simulink model "canrx_0x6A2"  (R2022b)
settings: configuration reference "SLDD_CFG" (kept outside this file)
values from neighbouring files (symbols this model uses):
  K_CAN_GMLAN_RX_DEFAULT_ANMSIG_VCM_CAN02 = 0.0    [canrx_0x6A2.sldd]
  K_CAN_GMLAN_RX_INVALID_SELECT = 0.0    [canrx_0x6A2.sldd]
  K_CAN_RQST_SEL_2 = 0.0    [canrx_0x6A2.sldd]
  K_RQST_DRCT_2 = 0.0    [canrx_0x6A2.sldd]
libraries: user_lib x1, simulink x1
settings Model: DataDictionary=canrx_0x6A2.sldd  Creator=Castiel  LastModifiedBy=Castiel
settings ConfigSetRef: SourceName=SLDD_CFG

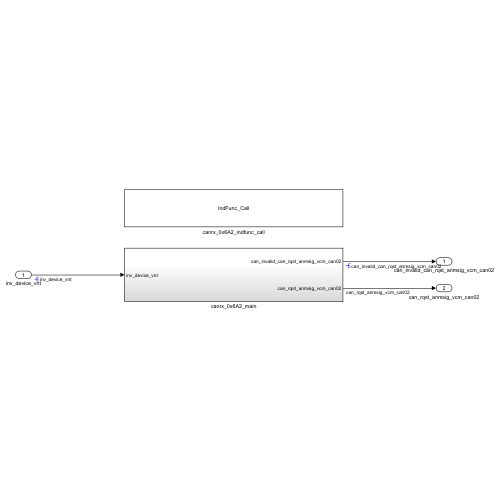
[thumbnail: Simulink's stored preview of the top-level diagram]
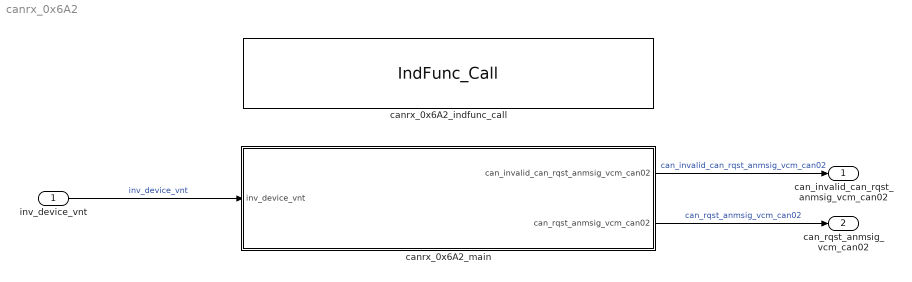
== system canrx_0x6A2 ==
  inv_device_vnt : Inport
  canrx_0x6A2_indfunc_call : user_lib/IndFunc_Call  siggroupIndex=Test  canid=6A2  signalTable={'UW','IFLayer_rx_anmsig_vcm_can02','SYCANC_COM2AP_6A2_rx_anmsig_vcm_can02'}  timeoutflag=off  extendid=off
      settings: SourceProductName=User Defined for IFLayer
  canrx_0x6A2_main : Subsystem
  can_invalid_can_rqst_anmsig_vcm_can02 : Outport
  can_rqst_anmsig_vcm_can02 : Outport  Port=2
  wires:
  inv_device_vnt/1 -> canrx_0x6A2_main/1(inv_device_vnt)  "inv_device_vnt"
  canrx_0x6A2_main/1(can_invalid_can_rqst_anmsig_vcm_can02) -> can_invalid_can_rqst_anmsig_vcm_can02/1  "can_invalid_can_rqst_anmsig_vcm_can02"
  canrx_0x6A2_main/2(can_rqst_anmsig_vcm_can02) -> can_rqst_anmsig_vcm_can02/1  "can_rqst_anmsig_vcm_can02"

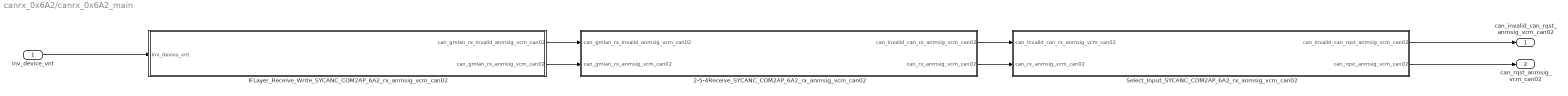
== system canrx_0x6A2/canrx_0x6A2_main ==
  inv_device_vnt : Inport
  2-5-4Receive_SYCANC_COM2AP_6A2_rx_anmsig_vcm_can02 : Subsystem  TreatAsAtomicUnit=on
      settings: RTWSystemCode=Nonreusable function
  IFLayer_Receive_Write_SYCANC_COM2AP_6A2_rx_anmsig_vcm_can02 : Subsystem  TreatAsAtomicUnit=on
      settings: RTWSystemCode=Nonreusable function
  Select_Input_SYCANC_COM2AP_6A2_rx_anmsig_vcm_can02 : Subsystem  TreatAsAtomicUnit=on
      settings: RTWSystemCode=Nonreusable function
  can_invalid_can_rqst_anmsig_vcm_can02 : Outport
  can_rqst_anmsig_vcm_can02 : Outport  Port=2
  wires:
  IFLayer_Receive_Write_SYCANC_COM2AP_6A2_rx_anmsig_vcm_can02/2(can_gmlan_rx_anmsig_vcm_can02) -> 2-5-4Receive_SYCANC_COM2AP_6A2_rx_anmsig_vcm_can02/2(can_gmlan_rx_anmsig_vcm_can02)
  IFLayer_Receive_Write_SYCANC_COM2AP_6A2_rx_anmsig_vcm_can02/1(can_gmlan_rx_invalid_anmsig_vcm_can02) -> 2-5-4Receive_SYCANC_COM2AP_6A2_rx_anmsig_vcm_can02/1(can_gmlan_rx_invalid_anmsig_vcm_can02)
  2-5-4Receive_SYCANC_COM2AP_6A2_rx_anmsig_vcm_can02/1(can_invalid_can_rx_anmsig_vcm_can02) -> Select_Input_SYCANC_COM2AP_6A2_rx_anmsig_vcm_can02/1(can_invalid_can_rx_anmsig_vcm_can02)
  2-5-4Receive_SYCANC_COM2AP_6A2_rx_anmsig_vcm_can02/2(can_rx_anmsig_vcm_can02) -> Select_Input_SYCANC_COM2AP_6A2_rx_anmsig_vcm_can02/2(can_rx_anmsig_vcm_can02)
  inv_device_vnt/1 -> IFLayer_Receive_Write_SYCANC_COM2AP_6A2_rx_anmsig_vcm_can02/1(inv_device_vnt)
  Select_Input_SYCANC_COM2AP_6A2_rx_anmsig_vcm_can02/1(can_invalid_can_rqst_anmsig_vcm_can02) -> can_invalid_can_rqst_anmsig_vcm_can02/1
  Select_Input_SYCANC_COM2AP_6A2_rx_anmsig_vcm_can02/2(can_rqst_anmsig_vcm_can02) -> can_rqst_anmsig_vcm_can02/1

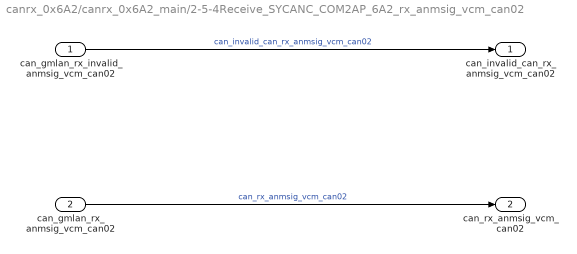
== system canrx_0x6A2/canrx_0x6A2_main/2-5-4Receive_SYCANC_COM2AP_6A2_rx_anmsig_vcm_can02 ==
  can_gmlan_rx_invalid_anmsig_vcm_can02 : Inport
  can_gmlan_rx_anmsig_vcm_can02 : Inport  Port=2
  can_invalid_can_rx_anmsig_vcm_can02 : Outport
  can_rx_anmsig_vcm_can02 : Outport  Port=2
  wires:
  can_gmlan_rx_anmsig_vcm_can02/1 -> can_rx_anmsig_vcm_can02/1  "can_rx_anmsig_vcm_can02"
  can_gmlan_rx_invalid_anmsig_vcm_can02/1 -> can_invalid_can_rx_anmsig_vcm_can02/1  "can_invalid_can_rx_anmsig_vcm_can02"

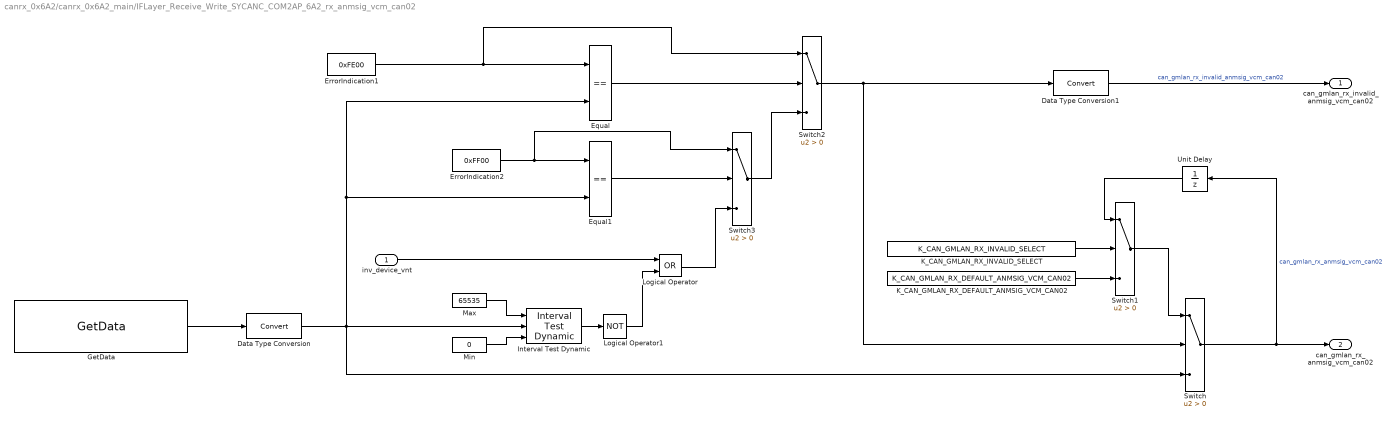
== system canrx_0x6A2/canrx_0x6A2_main/IFLayer_Receive_Write_SYCANC_COM2AP_6A2_rx_anmsig_vcm_can02 ==
  inv_device_vnt : Inport
  Data Type Conversion : DataTypeConversion  ConvertRealWorld=Stored Integer (SI)  SaturateOnIntegerOverflow=off  RndMeth=Floor
  Data Type Conversion1 : DataTypeConversion  ConvertRealWorld=Stored Integer (SI)  SaturateOnIntegerOverflow=off  RndMeth=Floor
  Equal : RelationalOperator  Operator===  OutDataTypeStr=boolean  RndMeth=Simplest  InputSameDT=off
  Equal1 : RelationalOperator  Operator===  OutDataTypeStr=boolean  RndMeth=Simplest  InputSameDT=off
  ErrorIndication1 : Constant  Value=0xFE00  OutDataTypeStr=Inherit: Inherit via back propagation
  ErrorIndication2 : Constant  Value=0xFF00  OutDataTypeStr=Inherit: Inherit via back propagation
  GetData : S-Function  FunctionName=GetData  Parameters=interface,signalType  SFunctionDeploymentMode=off  EnableBusSupport=off  mask{interface=SYCANC_COM2AP_6A2_rx_anmsig_vcm_can02, signalType=UW}
      mask prompts: signalType "Signal Type"
      mask TypeOptions signalType: UB | SB | UW | SW | UD | SD
      mask DialogControl Container4 Prompt: Singal Parameter
      mask Display:
      | interfaceName = get_param(gcbh, "interface");
      | s = strcat(interfaceName);
      | disp(s);
  Interval Test Dynamic : simulink/Logic and Bit Operations/Interval Test Dynamic  IntervalClosedRight=on  IntervalClosedLeft=on  OutDataTypeStr=boolean
  K_CAN_GMLAN_RX_DEFAULT_ANMSIG_VCM_CAN02 : Constant  Value=K_CAN_GMLAN_RX_DEFAULT_ANMSIG_VCM_CAN02  OutDataTypeStr=Inherit: Inherit via back propagation
  K_CAN_GMLAN_RX_INVALID_SELECT : Constant  Value=K_CAN_GMLAN_RX_INVALID_SELECT  OutDataTypeStr=Inherit: Inherit via back propagation
  Logical Operator : Logic  Operator=OR  AllPortsSameDT=off  OutDataTypeStr=boolean
  Logical Operator1 : Logic  Operator=NOT  AllPortsSameDT=off  OutDataTypeStr=boolean
  Max : Constant  Value=65535  OutDataTypeStr=Inherit: Inherit via back propagation
  Min : Constant  Value=0  OutDataTypeStr=Inherit: Inherit via back propagation
  Switch{,1..3} (4 alike) : Switch  Criteria=u2 > Threshold  SaturateOnIntegerOverflow=off  InputSameDT=off
  Unit Delay : UnitDelay  SampleTime=-1  HasFrameUpgradeWarning=on
  can_gmlan_rx_invalid_anmsig_vcm_can02 : Outport
  can_gmlan_rx_anmsig_vcm_can02 : Outport  Port=2
  wires:
  Switch1/1 -> Switch/1
  Unit Delay/1 -> Switch1/1
  inv_device_vnt/1 -> Logical Operator/1
  K_CAN_GMLAN_RX_DEFAULT_ANMSIG_VCM_CAN02/1 -> Switch1/3
  Max/1 -> Interval Test Dynamic/1
  Min/1 -> Interval Test Dynamic/3
  Switch/1 -> Unit Delay/1, can_gmlan_rx_anmsig_vcm_can02/1  "can_gmlan_rx_anmsig_vcm_can02"
  K_CAN_GMLAN_RX_INVALID_SELECT/1 -> Switch1/2
  Data Type Conversion1/1 -> can_gmlan_rx_invalid_anmsig_vcm_can02/1  "can_gmlan_rx_invalid_anmsig_vcm_can02"
  Logical Operator1/1 -> Logical Operator/2
  Interval Test Dynamic/1 -> Logical Operator1/1
  Equal/1 -> Switch2/2
  Switch2/1 -> Data Type Conversion1/1, Switch/2
  GetData/1 -> Data Type Conversion/1
  Equal1/1 -> Switch3/2
  Logical Operator/1 -> Switch3/3
  Switch3/1 -> Switch2/3
  Data Type Conversion/1 -> Equal1/2, Equal/2, Interval Test Dynamic/2, Switch/3
  ErrorIndication1/1 -> Switch2/1, Equal/1
  ErrorIndication2/1 -> Switch3/1, Equal1/1

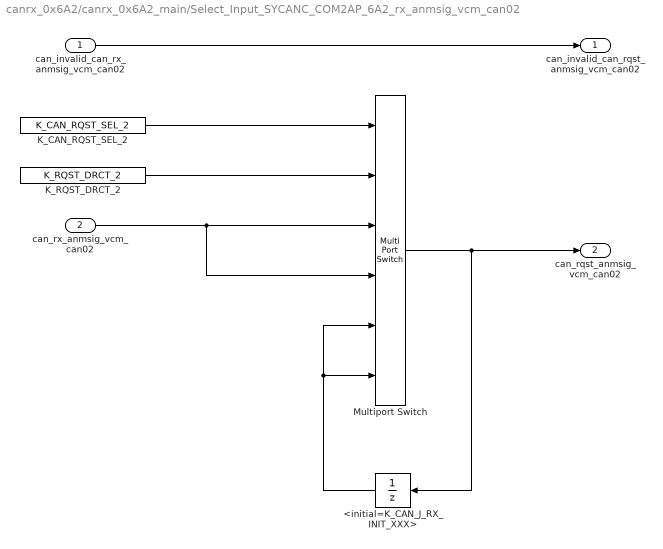
== system canrx_0x6A2/canrx_0x6A2_main/Select_Input_SYCANC_COM2AP_6A2_rx_anmsig_vcm_can02 ==
  can_invalid_can_rx_anmsig_vcm_can02 : Inport
  can_rx_anmsig_vcm_can02 : Inport  Port=2
  <initial=K_CAN_J_RX_INIT_XXX> : UnitDelay  SampleTime=-1  HasFrameUpgradeWarning=on
  K_CAN_RQST_SEL_2 : Constant  Value=K_CAN_RQST_SEL_2
  K_RQST_DRCT_2 : Constant  Value=K_RQST_DRCT_2
  Multiport Switch : MultiPortSwitch  DataPortOrder=Zero-based contiguous  Inputs=5  zeroidx=on  SaturateOnIntegerOverflow=off  InputSameDT=off
  can_invalid_can_rqst_anmsig_vcm_can02 : Outport
  can_rqst_anmsig_vcm_can02 : Outport  Port=2
  wires:
  K_CAN_RQST_SEL_2/1 -> Multiport Switch/1
  <initial=K_CAN_J_RX_INIT_XXX>/1 -> Multiport Switch/6, Multiport Switch/5
  Multiport Switch/1 -> can_rqst_anmsig_vcm_can02/1, <initial=K_CAN_J_RX_INIT_XXX>/1
  can_rx_anmsig_vcm_can02/1 -> Multiport Switch/4, Multiport Switch/3
  K_RQST_DRCT_2/1 -> Multiport Switch/2
  can_invalid_can_rx_anmsig_vcm_can02/1 -> can_invalid_can_rqst_anmsig_vcm_can02/1
